simulink model "Water_tankttemp"  (R2024a)
settings: Solver=VariableStepAuto  StartTime=0.0  StopTime=10.0  RelTol=1e-3
settings Model: Creator=Lenovo  LastModifiedBy=Lenovo

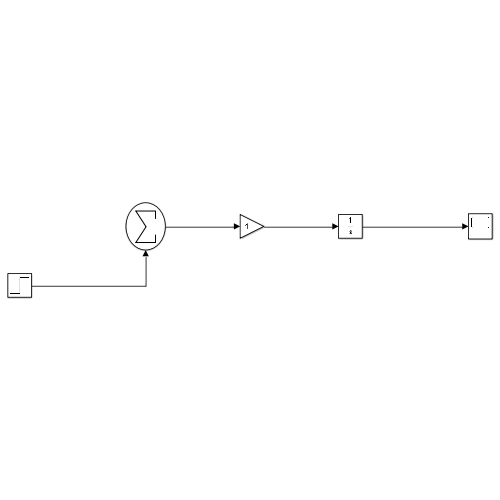
[thumbnail: Simulink's stored preview of the top-level diagram]
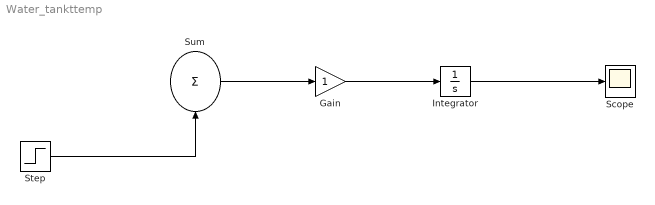
== system Water_tankttemp ==
  Gain : Gain
  Integrator : Integrator  InitialCondition=1
  Scope : Scope
  Step : Step  SampleTime=0
  Sum : Sum  Inputs=|+
  wires:
  Step/1 -> Sum/1
  Sum/1 -> Gain/1
  Gain/1 -> Integrator/1
  Integrator/1 -> Scope/1
